simulink model "behaelter1"  (Simulink 4.00)
settings: Solver=ode45  StartTime=0.0  StopTime=10.0  RelTol=1e-3
values from neighbouring files (symbols this model uses):
  AB = pi*(dB^2)/4    (= 0.0706858347058)    [behaelter_1.m]    (also in behaelter_2.m)
  AL = pi*(dL^2)/4    (= 0.00196349540849)    [behaelter_1.m]    (also in behaelter_2.m)
  D = 100    [behaelter_1.m]    (also in behaelter_2.m; mehrw_1.m = zeros(10,2); mehrw_2.m = zeros(10,2); mehrw_3.m = zeros(10,2))
  g = 9.81    [behaelter_1.m]    (also in behaelter_2.m; kette_1.m = 9.8; pendel_1.m = 9.8; pendel_2.m = 9.8)
  h0 = m0/(ro*AB)    (= 0.707355302631)    [behaelter_1.m]    (also in behaelter_2.m)
  m0 = 50    [behaelter_1.m]    (also in behaelter_2.m)
  r = 2    [behaelter_1.m]    (also in behaelter_2.m; mehrw_1.m = [0.05, 0.05, 0.05, 0.05, 0.05]; mehrw_2.m = [0.05, 0.05, 0.05, 0.05, 0.05]; mehrw_3.m = [0.05, 0.05, 0.05, 0.05, 0.05])
  ro = 1000    [behaelter_1.m]    (also in behaelter_2.m; kette_1.m = 10)
  x0 = 0.5    [behaelter_1.m]    (also in behaelter_2.m; kette_1.m = 1; mehrw_3.m = [0 0 0 0 0 1 0 0 0 0]; mehrw_4.m = [0 0 0 0 0 1 0 0 0 0])
settings Model: LastModifiedBy=Administrator  Refine=4  BlockReductionOpt=off

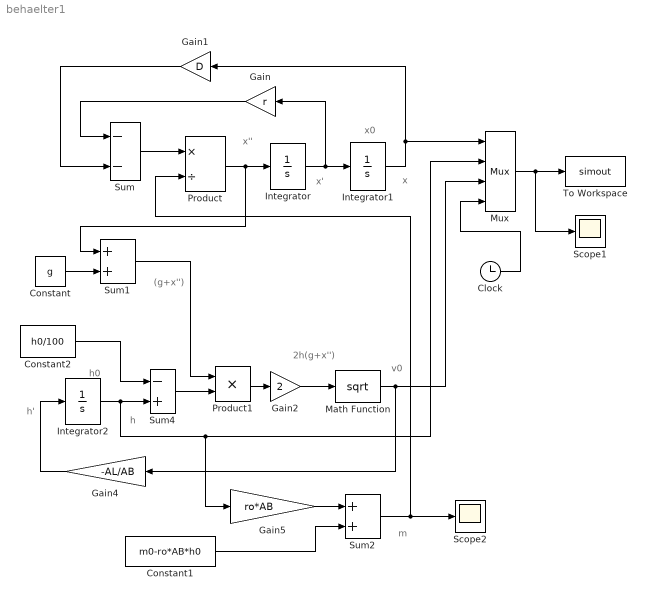
== system behaelter1 ==
  note: x
  note: x'
  note: x''
  note: x0
  note: v0
  note: (g+x'')
  note: h'
  note: h0
  note: h
  note: m
  note: 2h(g+x'')
  Clock : Clock
      settings: DisplayTime=off  Decimation=10
  Constant : Constant  Value=g
  Constant1 : Constant  Value=m0-ro*AB*h0
  Constant2 : Constant  Value=h0/100
  Gain : Gain  Orientation=left  Gain=r  Multiplication=Element-wise(K.*u)  SaturateOnIntegerOverflow=on
  Gain1 : Gain  Orientation=left  Gain=D  Multiplication=Element-wise(K.*u)  SaturateOnIntegerOverflow=on
  Gain2 : Gain  Gain=2  Multiplication=Element-wise(K.*u)  SaturateOnIntegerOverflow=on
  Gain4 : Gain  Orientation=left  Gain=-AL/AB  Multiplication=Element-wise(K.*u)  SaturateOnIntegerOverflow=on
  Gain5 : Gain  Gain=ro*AB  Multiplication=Element-wise(K.*u)  SaturateOnIntegerOverflow=on
  Integrator : Integrator  ExternalReset=none  InitialConditionSource=internal  InitialCondition=0  LimitOutput=off  UpperSaturationLimit=inf  LowerSaturationLimit=-inf  ShowSaturationPort=off  ShowStatePort=off  AbsoluteTolerance=auto
  Integrator1 : Integrator  ExternalReset=none  InitialConditionSource=internal  InitialCondition=x0  LimitOutput=off  UpperSaturationLimit=inf  LowerSaturationLimit=-inf  ShowSaturationPort=off  ShowStatePort=off  AbsoluteTolerance=auto
  Integrator2 : Integrator  ExternalReset=none  InitialConditionSource=internal  InitialCondition=h0  LimitOutput=on  UpperSaturationLimit=inf  LowerSaturationLimit=h0/100  ShowSaturationPort=off  ShowStatePort=off  AbsoluteTolerance=auto
  Math Function : Math  Operator=sqrt  OutputSignalType=real
  Mux : Mux  Inputs=4
      settings: DisplayOption=none
  Product : Product  Inputs=*/  Multiplication=Element-wise(.*)  SaturateOnIntegerOverflow=on
  Product1 : Product  Inputs=2  Multiplication=Element-wise(.*)  SaturateOnIntegerOverflow=on
  Scope1 : Scope
      settings: TimeRange=auto  YMin=-2.5  YMax=20  SaveToWorkspace=off  LimitDataPoints=on  MaxDataPoints=5000
  Scope2 : Scope
      settings: TimeRange=auto  YMin=0  YMax=50  SaveToWorkspace=off  SaveName=ScopeData2  LimitDataPoints=on  MaxDataPoints=5000
  Sum : Sum  Inputs=--  SaturateOnIntegerOverflow=on
  Sum1 : Sum  Inputs=++  SaturateOnIntegerOverflow=on
  Sum2 : Sum  Inputs=++  SaturateOnIntegerOverflow=on
  Sum4 : Sum  Inputs=-+  SaturateOnIntegerOverflow=on
  To Workspace : ToWorkspace  VariableName=simout  SampleTime=-1  SaveFormat=Array
  wires:
  Sum/1 -> Product/1
  Product/1 -> Integrator/1, Sum1/1
  Integrator/1 -> Integrator1/1, Gain/1
  Integrator1/1 -> Gain1/1, Mux/1
  Constant/1 -> Sum1/2
  Sum1/1 -> Product1/1
  Integrator2/1 -> Mux/2, Gain5/1, Sum4/2
  Product1/1 -> Gain2/1
  Gain2/1 -> Math Function/1
  Math Function/1 -> Mux/3, Gain4/1
  Gain4/1 -> Integrator2/1
  Mux/1 -> To Workspace/1, Scope1/1
  Gain/1 -> Sum/1
  Gain1/1 -> Sum/2
  Clock/1 -> Mux/4
  Sum2/1 -> Product/2, Scope2/1
  Gain5/1 -> Sum2/1
  Constant1/1 -> Sum2/2
  Constant2/1 -> Sum4/1
  Sum4/1 -> Product1/2
